simulink model "ya4"  (R2022b)
settings: Solver=VariableStepAuto  StartTime=0.0  StopTime=0.5  RelTol=1e-3
settings Model: Creator=Mahadevu Sudheer  LastModifiedBy=Mahadevu Sudheer

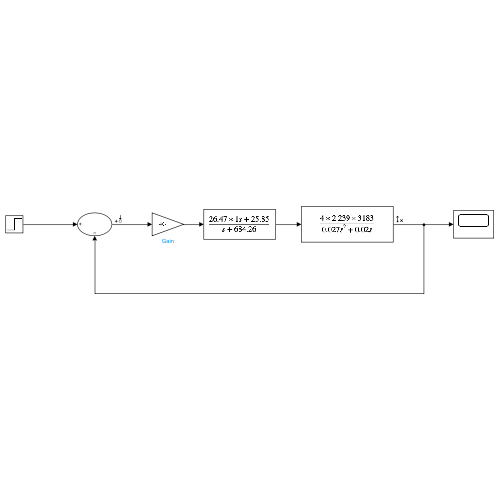
[thumbnail: Simulink's stored preview of the top-level diagram]
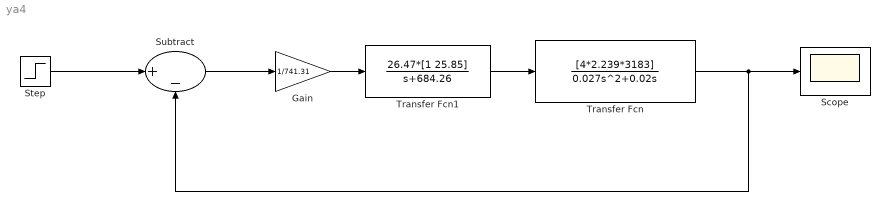
== system ya4 ==
  Gain : Gain  Gain=1/741.31
  Scope : Scope
  Step : Step  Time=0  SampleTime=0
  Subtract : Sum  Inputs=|+-
  Transfer Fcn : TransferFcn  Numerator=[4*2.239*3183]  Denominator=[0.027 0.02 0]
  Transfer Fcn1 : TransferFcn  Numerator=26.47*[1 25.85]  Denominator=[1 684.26]
  wires:
  Transfer Fcn1/1 -> Transfer Fcn/1
  Gain/1 -> Transfer Fcn1/1
  Subtract/1 -> Gain/1
  Step/1 -> Subtract/1
  Transfer Fcn/1 -> Subtract/2, Scope/1
